simulink model "Missile_Guidance"  (R2021b)
settings: Solver=ode4  StartTime=0.0  StopTime=40.0  FixedStep=0.01  RelTol=1e-3
values from neighbouring files (symbols this model uses):
  l_M0 = 80*pi/180    (= 1.3962634016)    [Initial_Conditions.m]
  N = 3    [Initial_Conditions.m]
  V_T = 600    [Initial_Conditions.m]
  X_M0 = 2000    [Initial_Conditions.m]
  X_T0 = 100    [Initial_Conditions.m]
  Z_M0 = 0    [Initial_Conditions.m]
  Z_T0 = 20000    [Initial_Conditions.m]
libraries: simulink x1
settings Model: Creator=SIVA RAO  LastModifiedBy=SIVA RAO

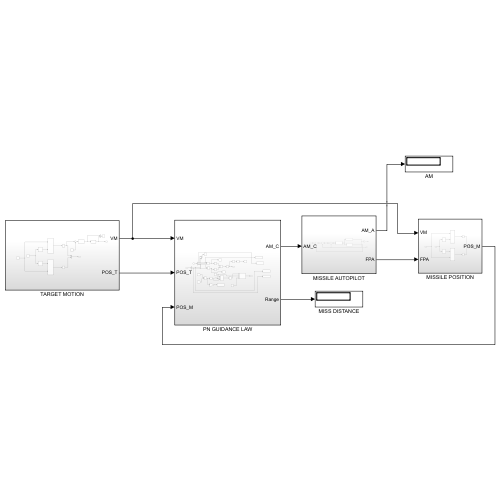
[thumbnail: Simulink's stored preview of the top-level diagram]
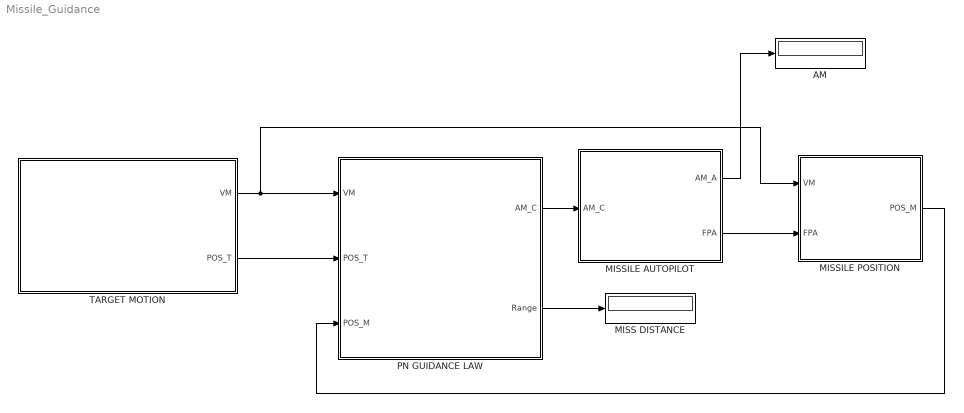
== system Missile_Guidance ==
  AM : Display
      settings: Format=bank
  MISS DISTANCE : Display
      settings: Format=bank
  MISSILE AUTOPILOT : Subsystem
  MISSILE POSITION : Subsystem
  PN GUIDANCE LAW : Subsystem
  TARGET MOTION : Subsystem
  wires:
  TARGET MOTION/2(POS_T) -> PN GUIDANCE LAW/2(POS_T)
  TARGET MOTION/1(VM) -> MISSILE POSITION/1(VM), PN GUIDANCE LAW/1(VM)
  MISSILE POSITION/1(POS_M) -> PN GUIDANCE LAW/3(POS_M)
  PN GUIDANCE LAW/1(AM_C) -> MISSILE AUTOPILOT/1(AM_C)
  MISSILE AUTOPILOT/2(FPA) -> MISSILE POSITION/2(FPA)
  MISSILE AUTOPILOT/1(AM_A) -> AM/1
  PN GUIDANCE LAW/2(Range) -> MISS DISTANCE/1

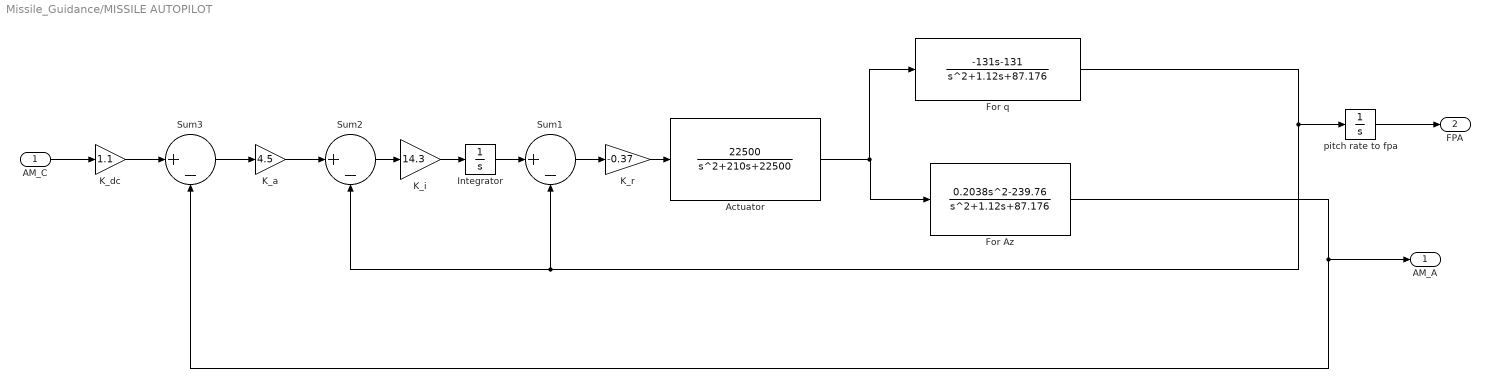
== system Missile_Guidance/MISSILE AUTOPILOT ==
  AM_C : Inport
  Actuator : TransferFcn  Numerator=[22500]  Denominator=[1 210 22500]
  For Az : TransferFcn  Numerator=[0.2038 0 -239.76]  Denominator=[1 1.12 87.176]
  For q : TransferFcn  Numerator=[-131 -131]  Denominator=[1 1.12 87.176]
  Integrator : Integrator
  K_a : Gain  Gain=4.5
  K_dc : Gain  Gain=1.1
  K_i : Gain  Gain=14.3
  K_r : Gain  Gain=-0.37
  Sum1 : Sum  Inputs=|+-
  Sum2 : Sum  Inputs=|+-
  Sum3 : Sum  Inputs=|+-
  pitch rate to fpa : Integrator  InitialCondition=l_M0
  AM_A : Outport
  FPA : Outport  Port=2
  wires:
  K_dc/1 -> Sum3/1
  K_a/1 -> Sum2/1
  K_i/1 -> Integrator/1
  K_r/1 -> Actuator/1
  Integrator/1 -> Sum1/1
  Actuator/1 -> For q/1, For Az/1
  For Az/1 -> AM_A/1, Sum3/2
  AM_C/1 -> K_dc/1
  For q/1 -> pitch rate to fpa/1, Sum2/2, Sum1/2
  Sum1/1 -> K_r/1
  Sum2/1 -> K_i/1
  Sum3/1 -> K_a/1
  pitch rate to fpa/1 -> FPA/1

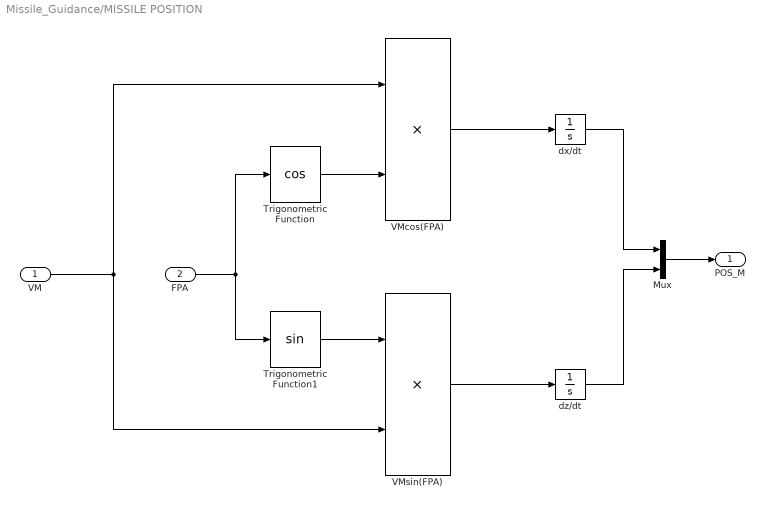
== system Missile_Guidance/MISSILE POSITION ==
  VM : Inport
  FPA : Inport  Port=2
  Mux : Mux  Inputs=2
  Trigonometric Function : Trigonometry  Operator=cos
  Trigonometric Function1 : Trigonometry
  VMcos(FPA) : Product
  VMsin(FPA) : Product
  dx/dt : Integrator  InitialCondition=X_M0
  dz/dt : Integrator  InitialCondition=Z_M0
  POS_M : Outport
  wires:
  VMsin(FPA)/1 -> dz/dt/1
  VMcos(FPA)/1 -> dx/dt/1
  Trigonometric Function/1 -> VMcos(FPA)/2
  FPA/1 -> Trigonometric Function1/1, Trigonometric Function/1
  Mux/1 -> POS_M/1
  VM/1 -> VMsin(FPA)/2, VMcos(FPA)/1
  dz/dt/1 -> Mux/2
  Trigonometric Function1/1 -> VMsin(FPA)/1
  dx/dt/1 -> Mux/1

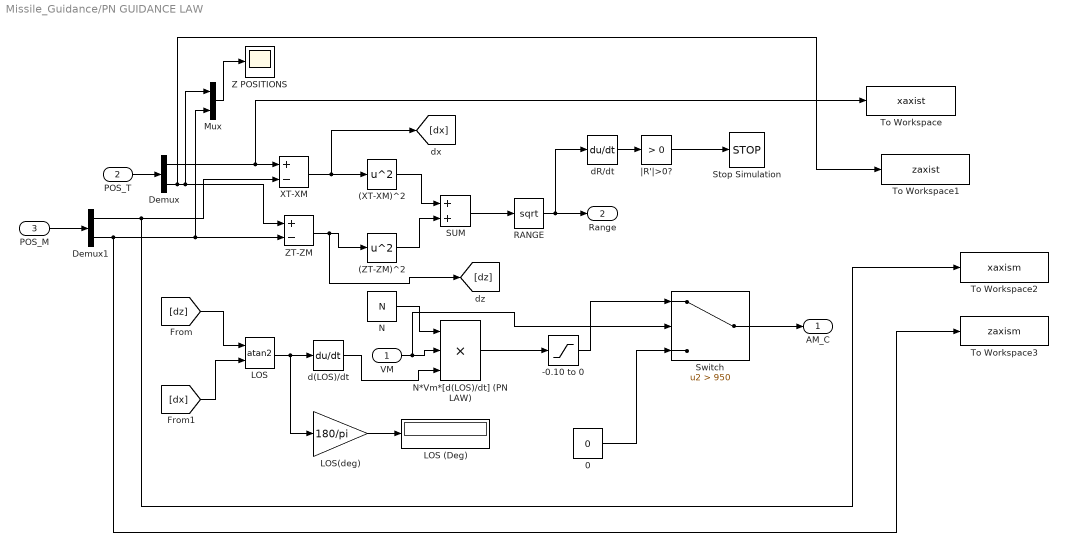
== system Missile_Guidance/PN GUIDANCE LAW ==
  VM : Inport
  POS_T : Inport  Port=2
  POS_M : Inport  Port=3
  (XT-XM)^2 : Math  Operator=square  SaturateOnIntegerOverflow=on
  (ZT-ZM)^2 : Math  Operator=square  SaturateOnIntegerOverflow=on
  -0.10 to 0 : Saturate  UpperLimit=0.0  LowerLimit=-0.10
  0 : Constant  Value=0
  Demux : Demux  Outputs=2
  Demux1 : Demux  Outputs=2
  LOS : Trigonometry  Operator=atan2
  LOS (Deg) : Display
  LOS(deg) : Gain  Gain=180/pi
  Mux : Mux  Inputs=2
  N : Constant  Value=N
  N*Vm*[d(LOS)/dt] (PN LAW) : Product  Inputs=3
  RANGE : Sqrt  SaturateOnIntegerOverflow=on
  SUM : Sum
  Stop Simulation : Stop
  Switch : Switch  Criteria=u2 > Threshold  Threshold=950
  To Workspace : ToWorkspace  VariableName=xaxist  SaveFormat=Timeseries  SampleTime=-1
  To Workspace1 : ToWorkspace  VariableName=zaxist  SaveFormat=Timeseries  SampleTime=-1
  To Workspace2 : ToWorkspace  VariableName=xaxism  SaveFormat=Timeseries  SampleTime=-1
  To Workspace3 : ToWorkspace  VariableName=zaxism  SaveFormat=Timeseries  SampleTime=-1
  XT-XM : Sum  Inputs=+-
  Z POSITIONS : Scope
  ZT-ZM : Sum  Inputs=+-
  d(LOS)/dt : Derivative
  dR/dt : Derivative
  |R'|>0? : simulink/Logic and Bit Operations/Compare To Zero  relop=>  OutDataTypeStr=boolean
  AM_C : Outport
  Range : Outport  Port=2
  wires:
  SUM/1 -> RANGE/1
  LOS(deg)/1 -> LOS (Deg)/1
  0/1 -> Switch/3
  LOS/1 -> LOS(deg)/1, d(LOS)/dt/1
  RANGE/1 -> Range/1, dR/dt/1
  Demux1/1 -> XT-XM/2, To Workspace2/1
  N*Vm*[d(LOS)/dt] (PN LAW)/1 -> -0.10 to 0/1
  Switch/1 -> AM_C/1
  Mux/1 -> Z POSITIONS/1
  Demux1/2 -> ZT-ZM/2, Mux/2, To Workspace3/1
  VM/1 -> Switch/2, N*Vm*[d(LOS)/dt] (PN LAW)/2
  Demux/2 -> To Workspace1/1, ZT-ZM/1, Mux/1
  ZT-ZM/1 -> [dz], (ZT-ZM)^2/1
  N/1 -> N*Vm*[d(LOS)/dt] (PN LAW)/1
  Demux/1 -> To Workspace/1, XT-XM/1
  d(LOS)/dt/1 -> N*Vm*[d(LOS)/dt] (PN LAW)/3
  XT-XM/1 -> [dx], (XT-XM)^2/1
  dR/dt/1 -> |R'|>0?/1
  [dz] -> LOS/1
  (ZT-ZM)^2/1 -> SUM/2
  |R'|>0?/1 -> Stop Simulation/1
  (XT-XM)^2/1 -> SUM/1
  POS_T/1 -> Demux/1
  POS_M/1 -> Demux1/1
  [dx] -> LOS/2
  -0.10 to 0/1 -> Switch/1

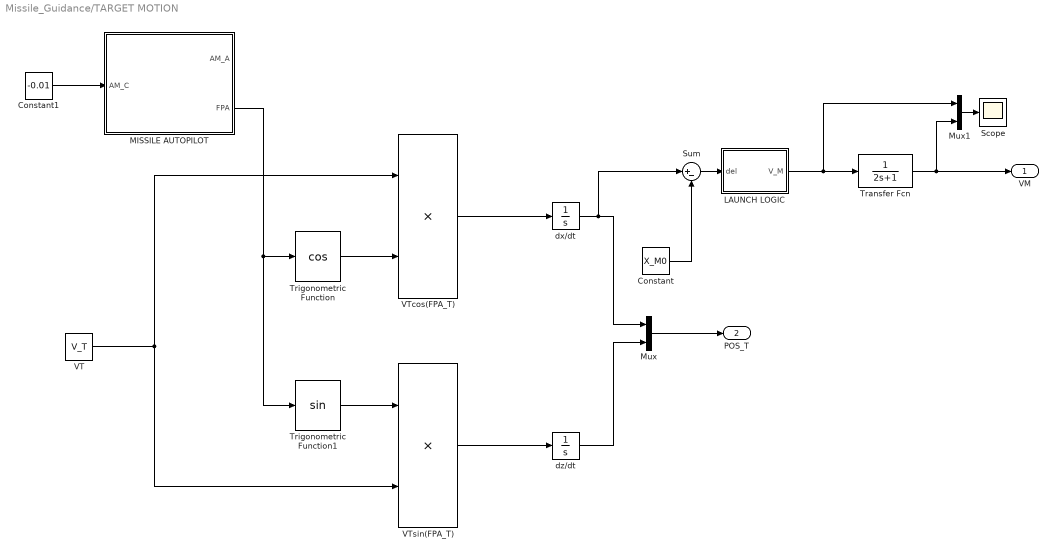
== system Missile_Guidance/TARGET MOTION ==
  Constant : Constant  Value=X_M0
  Constant1 : Constant  Value=-0.01
  LAUNCH LOGIC : MATLAB Function  TreatAsAtomicUnit=on
  MISSILE AUTOPILOT : Subsystem
  Mux : Mux  Inputs=2
  Mux1 : Mux  Inputs=2
  Scope : Scope
  Sum : Sum  Inputs=|+-
  Transfer Fcn : TransferFcn  Denominator=[2 1]
  Trigonometric Function : Trigonometry  Operator=cos
  Trigonometric Function1 : Trigonometry
  VT : Constant  Value=V_T
  VTcos(FPA_T) : Product
  VTsin(FPA_T) : Product
  dx/dt : Integrator  InitialCondition=X_T0
  dz/dt : Integrator  InitialCondition=Z_T0
  VM : Outport
  POS_T : Outport  Port=2
  wires:
  dx/dt/1 -> Sum/1, Mux/1
  Mux1/1 -> Scope/1
  LAUNCH LOGIC/1(V_M) -> Mux1/1, Transfer Fcn/1
  VTsin(FPA_T)/1 -> dz/dt/1
  Trigonometric Function1/1 -> VTsin(FPA_T)/1
  VT/1 -> VTsin(FPA_T)/2, VTcos(FPA_T)/1
  Trigonometric Function/1 -> VTcos(FPA_T)/2
  Sum/1 -> LAUNCH LOGIC/1(del)
  Transfer Fcn/1 -> VM/1, Mux1/2
  Constant/1 -> Sum/2
  VTcos(FPA_T)/1 -> dx/dt/1
  Mux/1 -> POS_T/1
  dz/dt/1 -> Mux/2
  MISSILE AUTOPILOT/2(FPA) -> Trigonometric Function1/1, Trigonometric Function/1
  Constant1/1 -> MISSILE AUTOPILOT/1(AM_C)

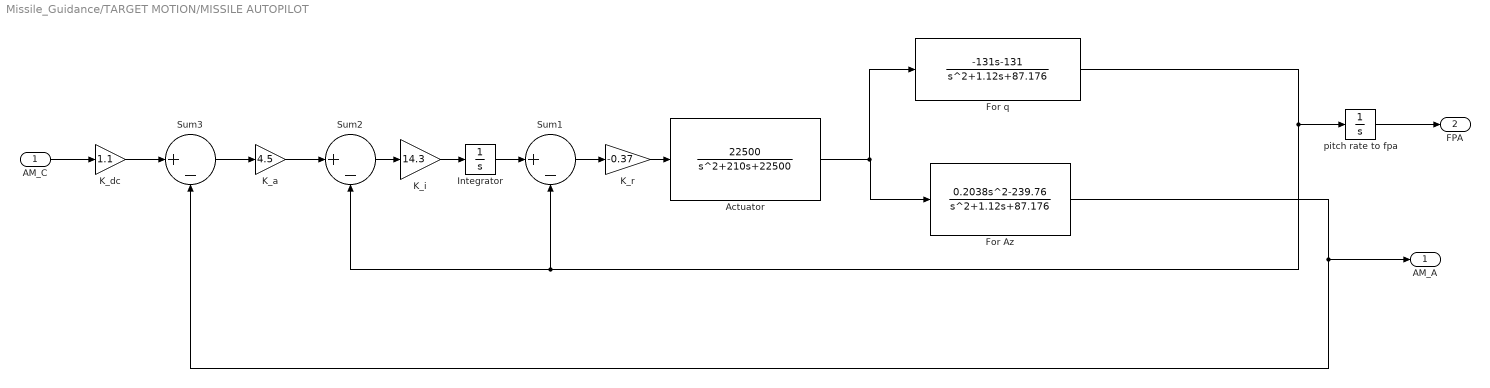
== system Missile_Guidance/TARGET MOTION/MISSILE AUTOPILOT ==
  AM_C : Inport
  Actuator : TransferFcn  Numerator=[22500]  Denominator=[1 210 22500]
  For Az : TransferFcn  Numerator=[0.2038 0 -239.76]  Denominator=[1 1.12 87.176]
  For q : TransferFcn  Numerator=[-131 -131]  Denominator=[1 1.12 87.176]
  Integrator : Integrator
  K_a : Gain  Gain=4.5
  K_dc : Gain  Gain=1.1
  K_i : Gain  Gain=14.3
  K_r : Gain  Gain=-0.37
  Sum1 : Sum  Inputs=|+-
  Sum2 : Sum  Inputs=|+-
  Sum3 : Sum  Inputs=|+-
  pitch rate to fpa : Integrator
  AM_A : Outport
  FPA : Outport  Port=2
  wires:
  K_dc/1 -> Sum3/1
  K_a/1 -> Sum2/1
  K_i/1 -> Integrator/1
  K_r/1 -> Actuator/1
  Integrator/1 -> Sum1/1
  Actuator/1 -> For q/1, For Az/1
  For Az/1 -> AM_A/1, Sum3/2
  AM_C/1 -> K_dc/1
  For q/1 -> pitch rate to fpa/1, Sum2/2, Sum1/2
  Sum1/1 -> K_r/1
  Sum2/1 -> K_i/1
  Sum3/1 -> K_a/1
  pitch rate to fpa/1 -> FPA/1

== matlab function Missile_Guidance/TARGET MOTION/LAUNCH LOGIC ==
  settings: updateMethod=DISCRETE
  data: del input; V_M output
function V_M = fcn(del)

persistent f
persistent Vel

if isempty(f)
    f=0;
end

if isempty(Vel)
    Vel=0;
end

if f==0 && del > -200
    f=1;
    Vel=1021;
end

V_M = Vel;

end
